simulink model "msdDoubleVectorizedSoln"  (R2020b)
settings: Solver=VariableStepAuto  StartTime=0.0  StopTime=20  RelTol=1e-6
settings Model: Creator=Rocksmithed  LastModifiedBy=Rocksmithed

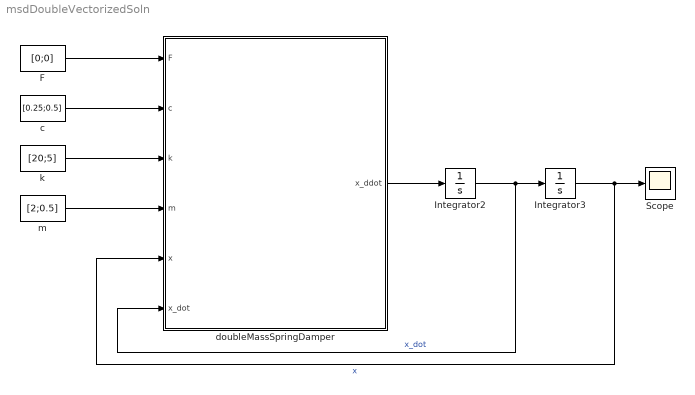
== system msdDoubleVectorizedSoln ==
  F : Constant  Value=[0;0]
  Integrator2 : Integrator  InitialCondition=[0;8]
  Integrator3 : Integrator  InitialCondition=[0;0]
  Scope : Scope
  c : Constant  Value=[0.25;0.5]
  doubleMassSpringDamper : MATLAB Function  TreatAsAtomicUnit=on
  k : Constant  Value=[20;5]
  m : Constant  Value=[2;0.5]
  wires:
  Integrator2/1 -> doubleMassSpringDamper/6(x_dot), Integrator3/1  "x_dot"
  Integrator3/1 -> doubleMassSpringDamper/5(x), Scope/1  "x"
  F/1 -> doubleMassSpringDamper/1(F)
  c/1 -> doubleMassSpringDamper/2(c)
  k/1 -> doubleMassSpringDamper/3(k)
  m/1 -> doubleMassSpringDamper/4(m)
  doubleMassSpringDamper/1(x_ddot) -> Integrator2/1

== matlab function msdDoubleVectorizedSoln/doubleMassSpringDamper ==
  data: F input; x_ddot output; c input; k input; m input; x input; x_dot input
function x_ddot = doubleMassSpringDamper(F, c, k, m, x, x_dot)
%#codegen

x_ddot = zeros(2,1);

x_ddot(1) = -(-F(1)+c(1).*x_dot(1)+k(1).*x(1)+c(2).*(x_dot(1)-x_dot(2))+k(2).*(x(1)-x(2)))./m(1);
x_ddot(2) = (F(2)+c(2).*(x_dot(1)-x_dot(2))+k(2).*(x(1)-x(2)))./m(2);
